simulink model "FrequencyModulation"  (R2020b)
settings: Solver=VariableStepAuto  StartTime=0.0  StopTime=20  RelTol=1e-3
undefined symbols (not defined in the file or in its folder): DiscIntNeverNeededParam
libraries: dsparch4 x1, commsynccomp2 x1
settings Model: Creator=Muthu  LastModifiedBy=Muthu

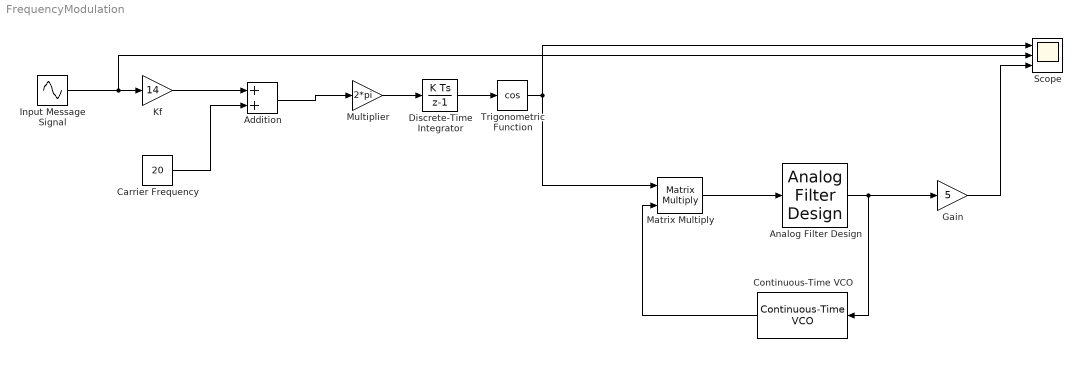
== system FrequencyModulation ==
  Addition : Sum
  Analog Filter Design : dsparch4/Analog Filter Design  method=Butterworth  filttype=Lowpass  N=3  Wlo=2  Whi=80  Rp=2  Rs=40
  Carrier Frequency : Constant  Value=20
  Continuous-Time VCO : commsynccomp2/Continuous-Time VCO  Ac=1  Fc=20  Kc=14/(2*pi)  Ph=pi/2
      settings: SourceProductBaseCode=CM
  Discrete-Time Integrator : DiscreteIntegrator  SampleTime=-1  ICPrevOutput=DiscIntNeverNeededParam  ICPrevScaledInput=DiscIntNeverNeededParam
  Gain : Gain  Gain=5
  Input Message Signal : Sin  Frequency=2  SampleTime=0.001
  Kf : Gain  Gain=14
  Matrix Multiply : Product  Multiplication=Matrix(*)
  Multiplier : Gain  Gain=2*pi
  Scope : Scope  NumInputPorts=3
  Trigonometric Function : Trigonometry  Operator=cos
  wires:
  Input Message Signal/1 -> Scope/2, Kf/1
  Kf/1 -> Addition/1
  Carrier Frequency/1 -> Addition/2
  Addition/1 -> Multiplier/1
  Trigonometric Function/1 -> Scope/1, Matrix Multiply/1
  Multiplier/1 -> Discrete-Time Integrator/1
  Discrete-Time Integrator/1 -> Trigonometric Function/1
  Matrix Multiply/1 -> Analog Filter Design/1
  Analog Filter Design/1 -> Gain/1, Continuous-Time VCO/1
  Continuous-Time VCO/1 -> Matrix Multiply/2
  Gain/1 -> Scope/3
